simulink model "HeartV10"  (R2023b)
settings: Solver=VariableStepAuto  StartTime=0.0  StopTime=10.0  RelTol=1e-3
libraries: Libs_second x151
(part 1 of 2)
settings Model: Creator=wai484  LastModifiedBy=wai484

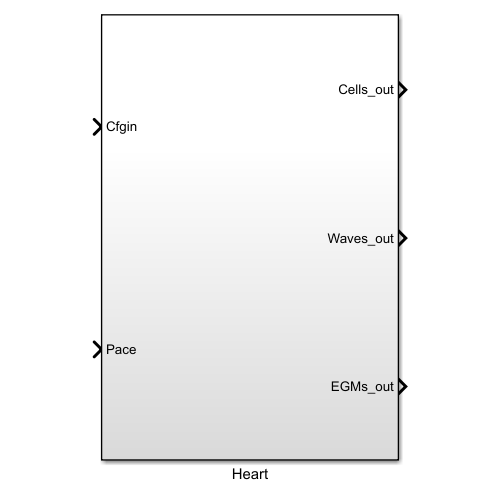
[thumbnail: Simulink's stored preview of the top-level diagram]
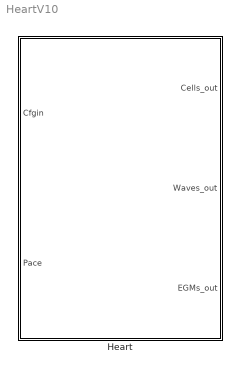
== system HeartV10 ==
  Heart : Subsystem
